simulink model "Mutant_9_of_purePursuitUSCityCopia"  (R2020a)
settings: Solver=FixedStepAuto  StartTime=0.0  StopTime=Ts  FixedStep=0.001  RelTol=1e-3
PreLoadFcn:
  | setUpPurePursuitUSCity
model workspace (MAT data in the model file):
  firstWarning = 0
  originalScenarioChecksum = 'F73A6DA3C723D3CA73A6F931B7A52A9C'
undefined symbols (not defined in the file): angVelGain, approximationReductionGain, L, ld, magnitude, minimalSpeed, nominalSpeed, psi_1, psi_2, psi_o, slope_x1, slope_x2, slope_y1, slope_y2, x_1, x_2, X_o, xRef, y_1, y_2, Y_o, yRef
libraries: simulink x15, autolibutils x4, autolibshared x3, robotalgslib x1
(part 1 of 3)
settings Model: SimulationMode=accelerator  EnablePacing=on  PacingRate=1000  Creator=valakshe  LastModifiedBy=Eskola
settings DebuggingCC: UnderSpecifiedDimensionMsg=warning

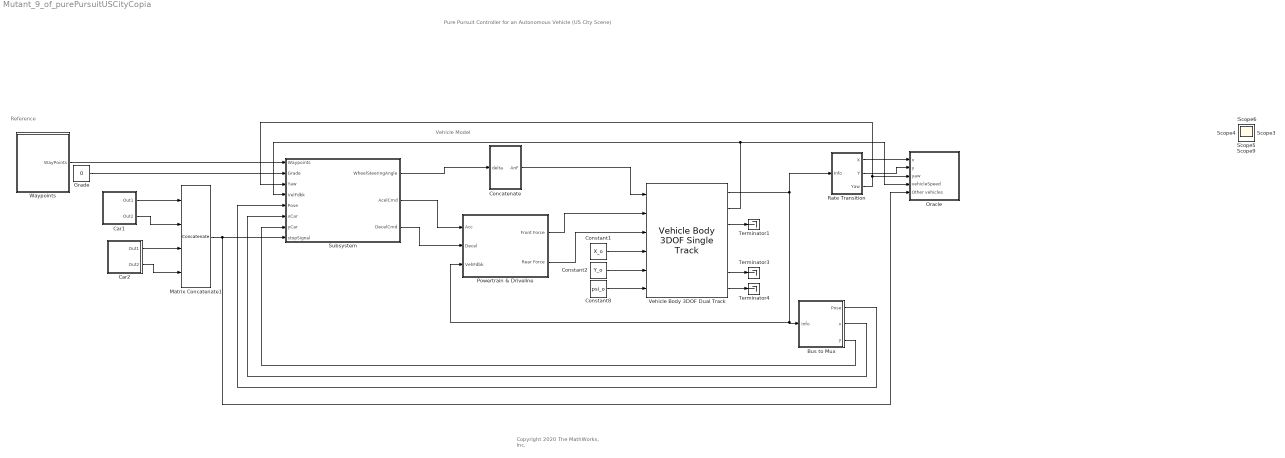
== system Mutant_9_of_purePursuitUSCityCopia ==
  note: Pure Pursuit Controller for an Autonomous Vehicle
      | (US City Scene)
  note: Copyright 2020 The MathWorks, Inc.
  note: Reference
  note: Vehicle Model
  Bus to Mux : Subsystem
  Car1 : Subsystem
  Car2 : Subsystem
  Concatenate : Subsystem
  Constant1 : Constant  Value=X_o
  Constant2 : Constant  Value=Y_o
  Constant8 : Constant  Value=psi_o
  Grade : Constant  Value=0
  Matrix Concatenate1 : Concatenate  NumInputs=4  Mode=Multidimensional array  ConcatenateDimension=2
  Oracle : Subsystem
  Powertrain & Driveline : Subsystem
      mask Display: image('vdbslibpt.png');
  Rate Transition : Subsystem
  Subsystem : Subsystem
  Terminator1 : Terminator
  Terminator3 : Terminator
  Terminator4 : Terminator
  Vehicle Body 3DOF Dual Track : autolibshared/Vehicle Body 3DOF Single Track  trackMode=Dual  inputMode=External longitudinal forces  frontSteerMode=on  rearSteerMode=off  windMode=off  muMode=off  extFMode=off  extMMode=off  extXo=on  extpsio=on  extxdoto=off  extro=off  extYo=on  extTamb=off  extydoto=off  aMode=2  NF=2  NR=2  m=2000  a=1.4  b=1.6  h=0.35  X_o=0  xdot_o=0  CalphaMode=off  sigmaMode=on  d=0  w=[1.4,1.4]  Cy_f=12e3  Cy_r=11e3  sigma_f=.1  sigma_r=.1  alpha_f_brk=[-.1 .1]  Cy_f_data=[-9e3 9e3]  alpha_r_brk=[-.1 .1]  Cy_r_data=[-9e3 9e3]  Y_o=0  ydot_o=0  Izz=4000  psi_o=0  r_o=0  Af=2  Cd=.3  Cl=.1  Cpm=.1  beta_w=[0:0.01:0.3]  Cs=[0:0.03:0.9]  Cym=[0:0.01:0.3]  Pabs=101325  Tair=273  g=9.81  mu=1  xdot_tol=.01  Fznom=5000  Fxtire_sat=7e4  Fytire_sat=7e4  longOff=0  latOff=0  vertOff=0  wrapAng=off
      settings: SourceProductBaseCode=PW,MT,VE,VP
  Waypoints : Subsystem
  Scope{,1..6,9} (8 alike) : Scope
  wires:
  Vehicle Body 3DOF Dual Track/7 -> Terminator4/1
  Vehicle Body 3DOF Dual Track/3 -> Terminator1/1
  Constant1/1 -> Vehicle Body 3DOF Dual Track/4
  Vehicle Body 3DOF Dual Track/6 -> Terminator3/1
  Constant2/1 -> Vehicle Body 3DOF Dual Track/5
  Concatenate/1(AnF) -> Vehicle Body 3DOF Dual Track/1
  Powertrain & Driveline/1(Front Force) -> Vehicle Body 3DOF Dual Track/2
  Powertrain & Driveline/2(Rear Force) -> Vehicle Body 3DOF Dual Track/3
  Constant8/1 -> Vehicle Body 3DOF Dual Track/6
  Vehicle Body 3DOF Dual Track/1 -> Rate Transition/1(Info), Powertrain & Driveline/3(VehFdbk), Bus to Mux/1(Info)
  Rate Transition/1(X) -> Oracle/1(x)
  Rate Transition/2(Y) -> Oracle/2(y)
  Rate Transition/3(Yaw) -> Subsystem/3(Yaw), Oracle/3(yaw)
  Car1/2(Out2) -> Matrix Concatenate1/2
  Car2/1(Out1) -> Matrix Concatenate1/3
  Car2/2(Out2) -> Matrix Concatenate1/4
  Car1/1(Out1) -> Matrix Concatenate1/1
  Waypoints/1(WayPoints) -> Subsystem/1(Waypoints)
  Grade/1 -> Subsystem/2(Grade)
  Vehicle Body 3DOF Dual Track/2 -> Oracle/4(vehicleSpeed), Subsystem/4(VelFdbk)
  Bus to Mux/1(Pose) -> Subsystem/5(Pose)
  Bus to Mux/2(x) -> Subsystem/6(xCar)
  Bus to Mux/3(y) -> Subsystem/7(yCar)
  Matrix Concatenate1/1 -> Oracle/5(Other vehicles), Subsystem/8(stopSignal)
  Subsystem/1(WheelSteeringAngle) -> Concatenate/1(delta)
  Subsystem/2(AcelCmd) -> Powertrain & Driveline/1(Acc)
  Subsystem/3(DecelCmd) -> Powertrain & Driveline/2(Decel)

== system Mutant_9_of_purePursuitUSCityCopia/Bus to Mux ==
  Info : Inport
  Bus Selector1 : BusSelector  OutputSignals=InertFrm.Cg.Disp.X,InertFrm.Cg.Disp.Y,InertFrm.Cg.Ang.psi
  Mux : Mux  Inputs=3
  Pose : Outport
  x : Outport  Port=2
  y : Outport  Port=3
  wires:
  Bus Selector1/3 -> Mux/3  "<psi>"
  Bus Selector1/1 -> Mux/1, x/1  "<X>"
  Mux/1 -> Pose/1
  Bus Selector1/2 -> y/1, Mux/2  "<Y>"
  Info/1 -> Bus Selector1/1

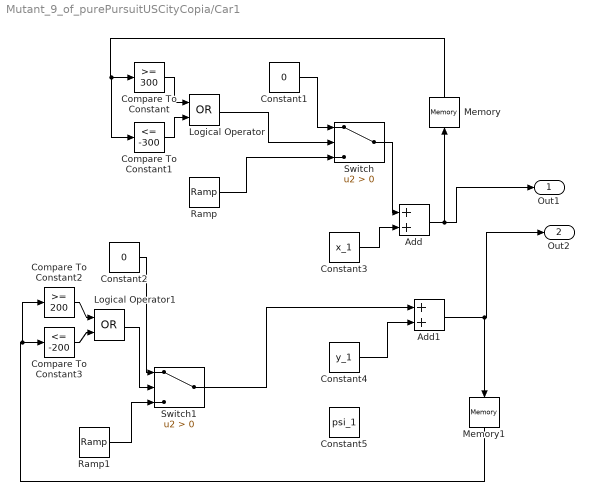
== system Mutant_9_of_purePursuitUSCityCopia/Car1 ==
  Add : Sum
  Add1 : Sum
  Compare To Constant : simulink/Logic and Bit Operations/Compare To Constant  relop=>=  const=300  OutDataTypeStr=boolean
  Compare To Constant1 : simulink/Logic and Bit Operations/Compare To Constant  relop=<=  const=-300  OutDataTypeStr=boolean
  Compare To Constant2 : simulink/Logic and Bit Operations/Compare To Constant  relop=>=  const=200  OutDataTypeStr=boolean
  Compare To Constant3 : simulink/Logic and Bit Operations/Compare To Constant  relop=<=  const=-200  OutDataTypeStr=boolean
  Constant1 : Constant  Value=0
  Constant2 : Constant  Value=0
  Constant3 : Constant  Value=x_1
  Constant4 : Constant  Value=y_1
  Constant5 : Constant  Value=psi_1
  Logical Operator : Logic  Operator=OR  AllPortsSameDT=off  OutDataTypeStr=boolean
  Logical Operator1 : Logic  Operator=OR  AllPortsSameDT=off  OutDataTypeStr=boolean
  Memory : Memory  InitialCondition=x_1
  Memory1 : Memory  InitialCondition=y_1
  Ramp : simulink/Sources/Ramp  slope=slope_x1  start=0  InitialOutput=0
  Ramp1 : simulink/Sources/Ramp  slope=slope_y1  start=0  InitialOutput=0
  Switch : Switch  Criteria=u2 > Threshold
  Switch1 : Switch  Criteria=u2 > Threshold
  Out1 : Outport
  Out2 : Outport  Port=2
  wires:
  Constant4/1 -> Add1/2
  Constant3/1 -> Add/2
  Add1/1 -> Memory1/1, Out2/1
  Add/1 -> Memory/1, Out1/1
  Ramp/1 -> Switch/3
  Constant1/1 -> Switch/1
  Switch/1 -> Add/1
  Compare To Constant/1 -> Logical Operator/1
  Compare To Constant1/1 -> Logical Operator/2
  Logical Operator/1 -> Switch/2
  Ramp1/1 -> Switch1/3
  Switch1/1 -> Add1/1
  Compare To Constant2/1 -> Logical Operator1/1
  Compare To Constant3/1 -> Logical Operator1/2
  Logical Operator1/1 -> Switch1/2
  Constant2/1 -> Switch1/1
  Memory/1 -> Compare To Constant1/1, Compare To Constant/1
  Memory1/1 -> Compare To Constant2/1, Compare To Constant3/1

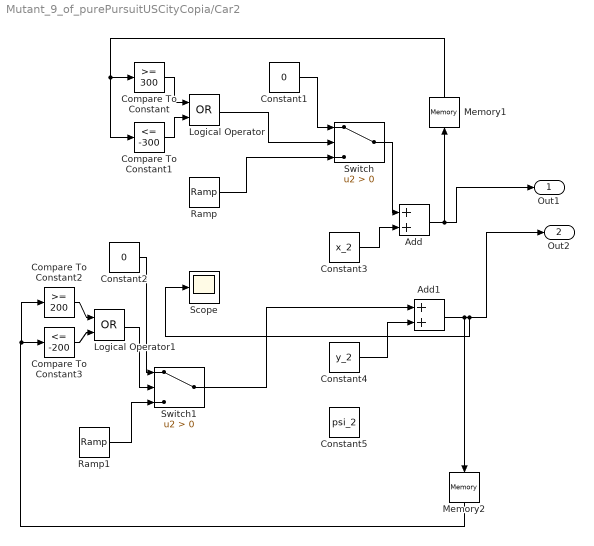
== system Mutant_9_of_purePursuitUSCityCopia/Car2 ==
  Add : Sum
  Add1 : Sum
  Compare To Constant : simulink/Logic and Bit Operations/Compare To Constant  relop=>=  const=300  OutDataTypeStr=boolean
  Compare To Constant1 : simulink/Logic and Bit Operations/Compare To Constant  relop=<=  const=-300  OutDataTypeStr=boolean
  Compare To Constant2 : simulink/Logic and Bit Operations/Compare To Constant  relop=>=  const=200  OutDataTypeStr=boolean
  Compare To Constant3 : simulink/Logic and Bit Operations/Compare To Constant  relop=<=  const=-200  OutDataTypeStr=boolean
  Constant1 : Constant  Value=0
  Constant2 : Constant  Value=0
  Constant3 : Constant  Value=x_2
  Constant4 : Constant  Value=y_2
  Constant5 : Constant  Value=psi_2
  Logical Operator : Logic  Operator=OR  AllPortsSameDT=off  OutDataTypeStr=boolean
  Logical Operator1 : Logic  Operator=OR  AllPortsSameDT=off  OutDataTypeStr=boolean
  Memory1 : Memory  InitialCondition=x_2
  Memory2 : Memory  InitialCondition=y_2
  Ramp : simulink/Sources/Ramp  slope=slope_x2  start=0  InitialOutput=0
  Ramp1 : simulink/Sources/Ramp  slope=slope_y2  start=0  InitialOutput=0
  Scope : Scope
  Switch : Switch  Criteria=u2 > Threshold
  Switch1 : Switch  Criteria=u2 > Threshold
  Out1 : Outport
  Out2 : Outport  Port=2
  wires:
  Constant2/1 -> Switch1/1
  Compare To Constant/1 -> Logical Operator/1
  Switch/1 -> Add/1
  Constant1/1 -> Switch/1
  Constant4/1 -> Add1/2
  Add/1 -> Memory1/1, Out1/1
  Logical Operator1/1 -> Switch1/2
  Add1/1 -> Out2/1, Scope/1, Memory2/1
  Logical Operator/1 -> Switch/2
  Compare To Constant1/1 -> Logical Operator/2
  Compare To Constant3/1 -> Logical Operator1/2
  Ramp/1 -> Switch/3
  Switch1/1 -> Add1/1
  Ramp1/1 -> Switch1/3
  Compare To Constant2/1 -> Logical Operator1/1
  Constant3/1 -> Add/2
  Memory1/1 -> Compare To Constant1/1, Compare To Constant/1
  Memory2/1 -> Compare To Constant2/1, Compare To Constant3/1

== system Mutant_9_of_purePursuitUSCityCopia/Concatenate ==
  delta : Inport
  Matrix Concatenate : Concatenate
  AnF : Outport  VectorParamsAs1DForOutWhenUnconnected=off
  tag scope: AnL=global, AnR=global
  wires:
  Matrix Concatenate/1 -> AnF/1
  delta/1 -> [AnL], [AnR], Matrix Concatenate/2, Matrix Concatenate/1

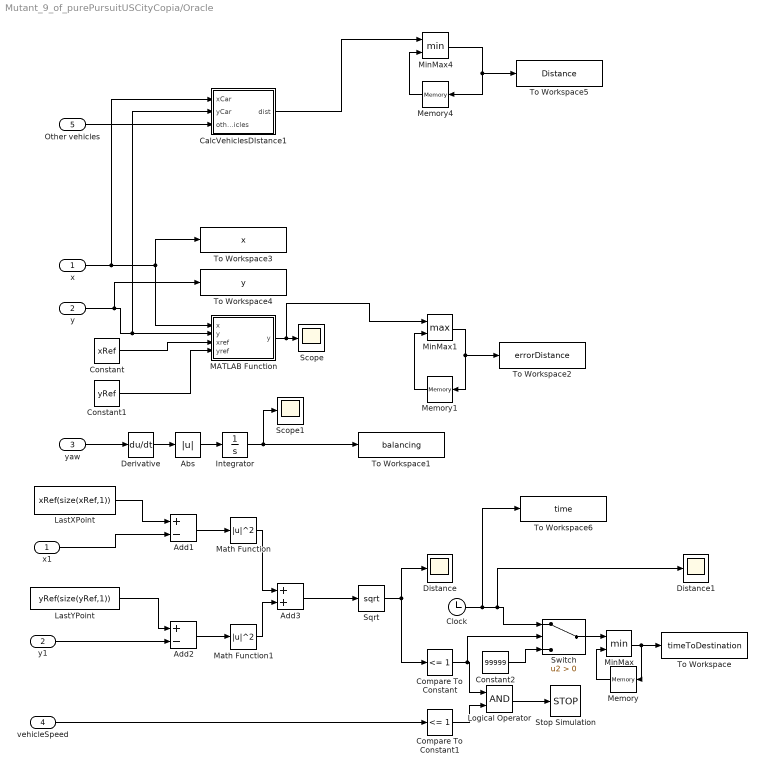
== system Mutant_9_of_purePursuitUSCityCopia/Oracle ==
  x : Inport
  y : Inport  Port=2
  yaw : Inport  Port=3
  vehicleSpeed : Inport  Port=4
  Other vehicles : Inport  Port=5
  Abs : Abs
  Add1 : Sum  Inputs=+-
  Add2 : Sum  Inputs=+-
  Add3 : Sum
  CalcVehiclesDIstance1 : MATLAB Function  TreatAsAtomicUnit=on
  Clock : Clock
  Compare To Constant : simulink/Logic and Bit Operations/Compare To Constant  relop=<=  const=1  OutDataTypeStr=boolean
  Compare To Constant1 : simulink/Logic and Bit Operations/Compare To Constant  relop=<=  const=1  OutDataTypeStr=boolean
  Constant : Constant  Value=xRef
  Constant1 : Constant  Value=yRef
  Constant2 : Constant  Value=99999
  Derivative : Derivative
  Distance : Scope
  Distance1 : Scope
  Integrator : Integrator
  LastXPoint : Constant  Value=xRef(size(xRef,1))  SampleTime=0.1
  LastYPoint : Constant  Value=yRef(size(yRef,1))  SampleTime=0.1
  Logical Operator : Logic  AllPortsSameDT=off  OutDataTypeStr=boolean
  MATLAB Function : MATLAB Function  TreatAsAtomicUnit=on
  Math Function : Math  Operator=magnitude^2  SaturateOnIntegerOverflow=on
  Math Function1 : Math  Operator=magnitude^2  SaturateOnIntegerOverflow=on
  Memory : Memory  InitialCondition=inf
  Memory1 : Memory
  Memory4 : Memory  InitialCondition=10000
  MinMax : MinMax  Inputs=2
  MinMax1 : MinMax  Function=max  Inputs=2
  MinMax4 : MinMax  Inputs=2
  Scope : Scope
  Scope1 : Scope
  Sqrt : Sqrt  SaturateOnIntegerOverflow=on
  Stop Simulation : Stop
  Switch : Switch  Criteria=u2 > Threshold
  To Workspace : ToWorkspace  VariableName=timeToDestination  SampleTime=-1
      settings: MaxDataPoints=1
  To Workspace1 : ToWorkspace  VariableName=balancing  SampleTime=-1
      settings: MaxDataPoints=1
  To Workspace2 : ToWorkspace  VariableName=errorDistance  SampleTime=-1
      settings: MaxDataPoints=1
  To Workspace3 : ToWorkspace  VariableName=x  SampleTime=-1
  To Workspace4 : ToWorkspace  VariableName=y  SampleTime=-1
  To Workspace5 : ToWorkspace  VariableName=Distance  SampleTime=-1
      settings: MaxDataPoints=1
  To Workspace6 : ToWorkspace  VariableName=time  SampleTime=-1
  x1 : InportShadow
  y1 : InportShadow  Port=2
  wires:
  Memory/1 -> MinMax/2
  Add3/1 -> Sqrt/1
  Integrator/1 -> To Workspace1/1, Scope1/1
  vehicleSpeed/1 -> Compare To Constant1/1
  Compare To Constant1/1 -> Logical Operator/2
  MinMax4/1 -> Memory4/1, To Workspace5/1
  Other vehicles/1 -> CalcVehiclesDIstance1/3(otherVehicles)
  Memory1/1 -> MinMax1/2
  MinMax1/1 -> To Workspace2/1, Memory1/1
  CalcVehiclesDIstance1/1(dist) -> MinMax4/1
  Memory4/1 -> MinMax4/2
  x1/1 -> Add1/2
  Clock/1 -> To Workspace6/1, Distance1/1, Switch/1
  Constant1/1 -> MATLAB Function/4(yref)
  Compare To Constant/1 -> Switch/2, Logical Operator/1
  MinMax/1 -> Memory/1, To Workspace/1
  y/1 -> To Workspace4/1, CalcVehiclesDIstance1/2(yCar), MATLAB Function/2("y ")
  Constant2/1 -> Switch/3
  Constant/1 -> MATLAB Function/3(xref)
  Add1/1 -> Math Function/1
  Add2/1 -> Math Function1/1
  LastYPoint/1 -> Add2/1
  Abs/1 -> Integrator/1
  LastXPoint/1 -> Add1/1
  MATLAB Function/1(y) -> MinMax1/1, Scope/1
  Math Function1/1 -> Add3/2
  y1/1 -> Add2/2
  Math Function/1 -> Add3/1
  Sqrt/1 -> Compare To Constant/1, Distance/1
  Derivative/1 -> Abs/1
  x/1 -> CalcVehiclesDIstance1/1(xCar), MATLAB Function/1(x), To Workspace3/1
  Switch/1 -> MinMax/1
  yaw/1 -> Derivative/1
  Logical Operator/1 -> Stop Simulation/1

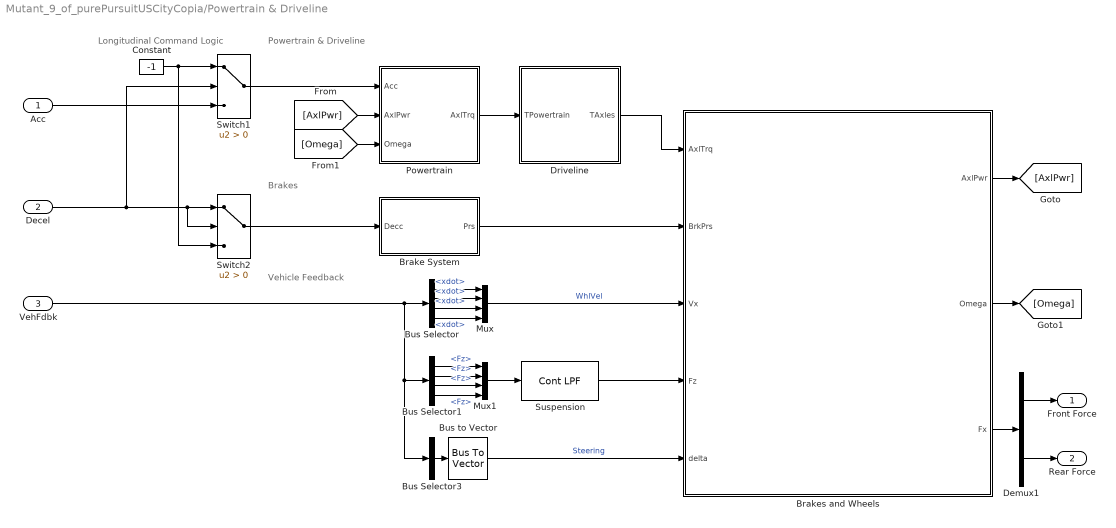
== system Mutant_9_of_purePursuitUSCityCopia/Powertrain & Driveline ==
  note: Vehicle Feedback
  note: Powertrain & Driveline
  note: Brakes
  note: Longitudinal Command Logic
  Acc : Inport
  Decel : Inport  Port=2
  VehFdbk : Inport  Port=3
  Brake System : Subsystem
  Brakes and Wheels : Subsystem  TreatAsAtomicUnit=on
      mask Display: image('vdbslibwhls.png');
  Bus Selector : BusSelector  OutputSignals=BdyFrm.FrntAxl.Lft.Vel.xdot,BdyFrm.FrntAxl.Rght.Vel.xdot,BdyFrm.RearAxl.Lft.Vel.xdot,BdyFrm.RearAxl.Rght.Vel.xdot
  Bus Selector1 : BusSelector  OutputSignals=BdyFrm.Forces.FrntAxl.Lft.Fz,BdyFrm.Forces.FrntAxl.Rght.Fz,BdyFrm.Forces.RearAxl.Lft.Fz,BdyFrm.Forces.RearAxl.Rght.Fz
  Bus Selector3 : BusSelector  OutputSignals=BdyFrm.FrntAxl.Steer.WhlAngFL,BdyFrm.FrntAxl.Steer.WhlAngFR,BdyFrm.RearAxl.Steer.WhlAngRL,BdyFrm.RearAxl.Steer.WhlAngRR  OutputAsBus=on
  Bus to Vector : BusToVector
  Constant : Constant  Value=-1
  Demux1 : Demux  Outputs=[2 2]
  Driveline : Subsystem  Variant=on  VariantControlMode=Label  VariantControl=Variant1  LabelModeActiveChoice=0
  Mux : Mux
  Mux1 : Mux
  Powertrain : Subsystem
  Suspension : autolibutils/Cont LPF  wc=10*pi*2  aMode=2
      settings: SourceProductBaseCode=PW,MT,AR,VE,VP
  Switch1 : Switch  Criteria=u2 > Threshold
  Switch2 : Switch  Criteria=u2 > Threshold
  Front Force : Outport  VectorParamsAs1DForOutWhenUnconnected=off
  Rear Force : Outport  Port=2  VectorParamsAs1DForOutWhenUnconnected=off
  wires:
  Brake System/1(Prs) -> Brakes and Wheels/2(BrkPrs)
  Switch2/1 -> Brake System/1(Decc)
  [Omega] -> Powertrain/3(Omega)
  [AxlPwr] -> Powertrain/2(AxlPwr)
  Brakes and Wheels/2(Omega) -> [Omega]
  Powertrain/1(AxlTrq) -> Driveline/1(TPowertrain)
  Switch1/1 -> Powertrain/1(Acc)
  Bus Selector1/4 -> Mux1/4  "<Fz>"
  Bus Selector1/3 -> Mux1/3  "<Fz>"
  Bus Selector1/2 -> Mux1/2  "<Fz>"
  Bus Selector1/1 -> Mux1/1  "<Fz>"
  Bus Selector/4 -> Mux/4  "<xdot>"
  Bus Selector/3 -> Mux/3  "<xdot>"
  Bus Selector/2 -> Mux/2  "<xdot>"
  Bus Selector/1 -> Mux/1  "<xdot>"
  Suspension/1 -> Brakes and Wheels/4(Fz)
  Mux1/1 -> Suspension/1
  Bus to Vector/1 -> Brakes and Wheels/5(delta)  "Steering"
  Bus Selector3/1 -> Bus to Vector/1
  Brakes and Wheels/3(Fx) -> Demux1/1
  Brakes and Wheels/1(AxlPwr) -> [AxlPwr]
  Driveline/1(TAxles) -> Brakes and Wheels/1(AxlTrq)
  Demux1/2 -> Rear Force/1
  Demux1/1 -> Front Force/1
  VehFdbk/1 -> Bus Selector/1, Bus Selector1/1, Bus Selector3/1
  Mux/1 -> Brakes and Wheels/3(Vx)  "WhlVel"
  Constant/1 -> Switch1/1, Switch2/3
  Acc/1 -> Switch1/3
  Decel/1 -> Switch2/1, Switch2/2, Switch1/2

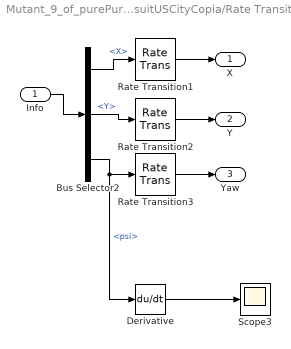
== system Mutant_9_of_purePursuitUSCityCopia/Rate Transition ==
  Info : Inport
  Bus Selector2 : BusSelector  OutputSignals=InertFrm.Geom.Disp.X,InertFrm.Geom.Disp.Y,InertFrm.Cg.Ang.psi
  Derivative : Derivative
  Rate Transition1 : RateTransition  InitialCondition=X_o  OutPortSampleTime=0.01
  Rate Transition2 : RateTransition  InitialCondition=Y_o  OutPortSampleTime=0.01
  Rate Transition3 : RateTransition  OutPortSampleTime=0.01
  Scope3 : Scope
  X : Outport
  Y : Outport  Port=2
  Yaw : Outport  Port=3
  wires:
  Info/1 -> Bus Selector2/1
  Rate Transition3/1 -> Yaw/1
  Rate Transition2/1 -> Y/1
  Rate Transition1/1 -> X/1
  Bus Selector2/1 -> Rate Transition1/1  "<X>"
  Bus Selector2/3 -> Derivative/1, Rate Transition3/1  "<psi>"
  Bus Selector2/2 -> Rate Transition2/1  "<Y>"
  Derivative/1 -> Scope3/1

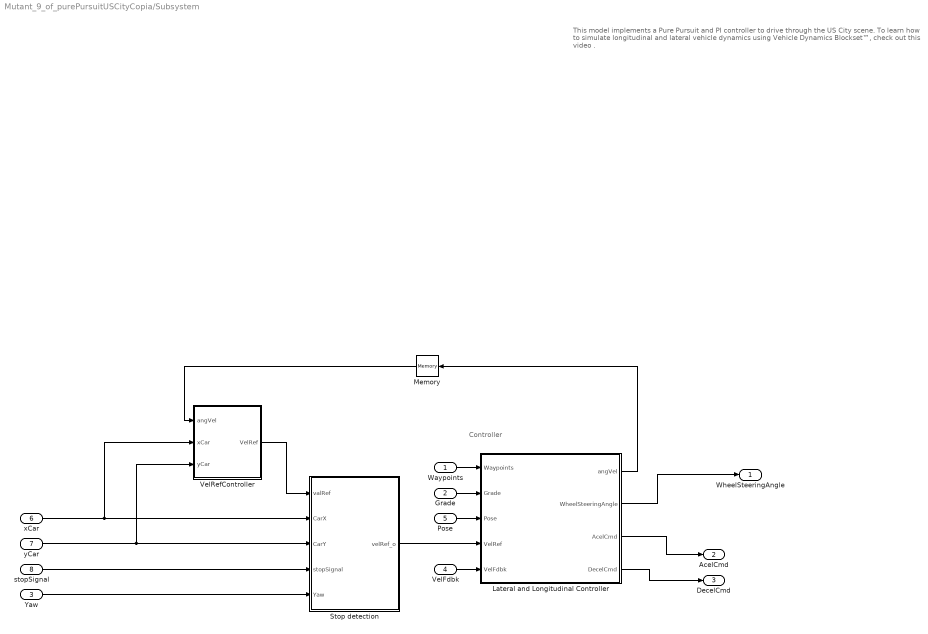
== system Mutant_9_of_purePursuitUSCityCopia/Subsystem ==
  note: This model implements a Pure Pursuit and PI controller to drive through the US City scene.
      | To learn how to simulate longitudinal and lateral vehicle dynamics using Vehicle Dynamics
      | Blockset™, check out this video .
  note: Controller
  Waypoints : Inport
  Grade : Inport  Port=2
  Yaw : Inport  Port=3
  VelFdbk : Inport  Port=4
  Pose : Inport  Port=5
  xCar : Inport  Port=6
  yCar : Inport  Port=7
  stopSignal : Inport  Port=8
  Lateral and Longitudinal Controller : Subsystem
  Memory : Memory
  Stop detection : Subsystem
  VelRefController : Subsystem
  WheelSteeringAngle : Outport
  AcelCmd : Outport  Port=2
  DecelCmd : Outport  Port=3
  wires:
  xCar/1 -> VelRefController/2(xCar), Stop detection/2(CarX)
  VelRefController/1(VelRef) -> Stop detection/1(valRef)
  VelFdbk/1 -> Lateral and Longitudinal Controller/5(VelFdbk)
  Lateral and Longitudinal Controller/1(angVel) -> Memory/1
  Lateral and Longitudinal Controller/3(AcelCmd) -> AcelCmd/1
  Stop detection/1(velRef_o) -> Lateral and Longitudinal Controller/4(VelRef)
  Waypoints/1 -> Lateral and Longitudinal Controller/1(Waypoints)
  yCar/1 -> Stop detection/3(CarY), VelRefController/3(yCar)
  Memory/1 -> VelRefController/1(angVel)
  Lateral and Longitudinal Controller/2(WheelSteeringAngle) -> WheelSteeringAngle/1
  Yaw/1 -> Stop detection/5(Yaw)
  Pose/1 -> Lateral and Longitudinal Controller/3(Pose)
  Lateral and Longitudinal Controller/4(DecelCmd) -> DecelCmd/1
  Grade/1 -> Lateral and Longitudinal Controller/2(Grade)
  stopSignal/1 -> Stop detection/4(stopSignal)

== system Mutant_9_of_purePursuitUSCityCopia/Waypoints ==
  Constant3 : Constant  Value=xRef  SampleTime=0.1
  Constant4 : Constant  Value=yRef  SampleTime=0.1
  Matrix Concatenate : Concatenate  Mode=Multidimensional array  ConcatenateDimension=2
  WayPoints : Outport
  wires:
  Constant4/1 -> Matrix Concatenate/2
  Constant3/1 -> Matrix Concatenate/1
  Matrix Concatenate/1 -> WayPoints/1

== system Mutant_9_of_purePursuitUSCityCopia/Powertrain & Driveline/Brake System ==
  Decc : Inport
  Hydraulics : autolibutils/Cont LPF  wc=30*pi*2  aMode=2
      settings: SourceProductBaseCode=PW,MT,AR,VE,VP
  Pressure : Gain  Gain=2e7
  Saturation1 : Saturate  UpperLimit=inf  LowerLimit=0  ZeroCross=off
  Selector : Selector  InputPortWidth=1  IndexOptions=Index vector (dialog)  Indices=[1 1 1 1]  OutputSizes=1
  Signal Specification : SignalSpecification  Unit=Pa
  Prs : Outport  VectorParamsAs1DForOutWhenUnconnected=off
  wires:
  Signal Specification/1 -> Prs/1
  Decc/1 -> Saturation1/1
  Selector/1 -> Signal Specification/1
  Saturation1/1 -> Hydraulics/1
  Hydraulics/1 -> Pressure/1
  Pressure/1 -> Selector/1
